simulink model "Hornet_6DOF_FlightSim"  (R2026b)
settings: Solver=VariableStepAuto  StopTime=25.0
values from neighbouring files (symbols this model uses):
  F_g_I = [-weight;0;0]    [Hornet_6DOF_FS_init.m]
  g = 9.81    [Hornet_6DOF_FS_init.m]    (also in hornet_sim_1D_init.m)
  gimbal_max = deg2rad(8)    [Hornet_6DOF_FS_init.m]
  I = [1 0 0 ... (first row only)    [Hornet_6DOF_FS_init.m]
  L_EDF = 1    [Hornet_6DOF_FS_init.m]
  m = 100    [Hornet_6DOF_FS_init.m]    (also in hornet_sim_1D_init.m = 2)
  PID_KD_pitch = 4.0    (= 4)    [Hornet_6DOF_FS_init.m]
  PID_KD_yaw = 4.0    (= 4)    [Hornet_6DOF_FS_init.m]
  PID_KI_pitch = 0.0    (= 0)    [Hornet_6DOF_FS_init.m]
  PID_KI_yaw = 0.0    (= 0)    [Hornet_6DOF_FS_init.m]
  PID_KP_pitch = 4.0    (= 4)    [Hornet_6DOF_FS_init.m]
  PID_KP_yaw = 4.0    (= 4)    [Hornet_6DOF_FS_init.m]
  PIDX_KD_pos = 0.0    (= 0)    [Hornet_6DOF_FS_init.m]
  PIDX_KI_pos = 0.0    (= 0)    [Hornet_6DOF_FS_init.m]
  PIDX_KP_pos = 0.0    (= 0)    [Hornet_6DOF_FS_init.m]
  PIDY_KD_pos = 0.6    [Hornet_6DOF_FS_init.m]
  PIDY_KI_pos = 0.0    (= 0)    [Hornet_6DOF_FS_init.m]
  PIDY_KP_pos = 0.2    [Hornet_6DOF_FS_init.m]
  PIDZ_KD_pos = 0.05    [Hornet_6DOF_FS_init.m]
  PIDZ_KD_vel = 0.0    (= 0)    [Hornet_6DOF_FS_init.m]
  PIDZ_KI_pos = 0.0    (= 0)    [Hornet_6DOF_FS_init.m]
  PIDZ_KI_vel = 0.0    (= 0)    [Hornet_6DOF_FS_init.m]
  PIDZ_KP_pos = 0.4    [Hornet_6DOF_FS_init.m]
  PIDZ_KP_vel = 1.0    (= 1)    [Hornet_6DOF_FS_init.m]
  Position_Target_inertial = [x_targ; y_targ;z_targ]    [Hornet_6DOF_FS_init.m]
  vx0 = 0    [Hornet_6DOF_FS_init.m]    (also in hornet_sim_1D_init.m)
  vy0 = 0    [Hornet_6DOF_FS_init.m]
  vz0 = 0    [Hornet_6DOF_FS_init.m]
  x0 = 0    [Hornet_6DOF_FS_init.m]    (also in hornet_sim_1D_init.m = 1)
  x_hat_body = [1;0;0]    [Hornet_6DOF_FS_init.m]
  y0 = 0    [Hornet_6DOF_FS_init.m]
  z0 = 0    [Hornet_6DOF_FS_init.m]
undefined symbols (not defined in the file or in its folder): DiscIntNeverNeededParam
libraries: slpidlib x5, matrix_library x1, sharedutil x1, aerolibutil x1
settings Model: Creator=11and  LastModifiedBy=jet
settings RTWCC: GenCodeOnly=on
settings SimscapeCC: SimscapeLogType=all  SimscapeNominalValues="[{\"value\":\"1\",\"unit\":\"A\"},{\"value\":\"1\",\"unit\":\"bar\"},{\"value\":\"1\",\"unit\":\"cm^2\"},{\"value\":\"1\",\"unit\":\"cm^3/s\"},{\"value\":\"1\",\"unit\":\"kJ/kg\"},{\"value\":\"1\",\"unit\":\"kW\"},{\"value\":\"1\",\"unit\":\"l\"},{\"value\":\"1\",\"unit\":\"N\"},{\"value\":\"1\",\"unit\":\"N*m\"},{\"value\":\"1\",\"unit\":\"V\"},{\"value\":\"0.001\",\"unit\":\"Wb\"}]"

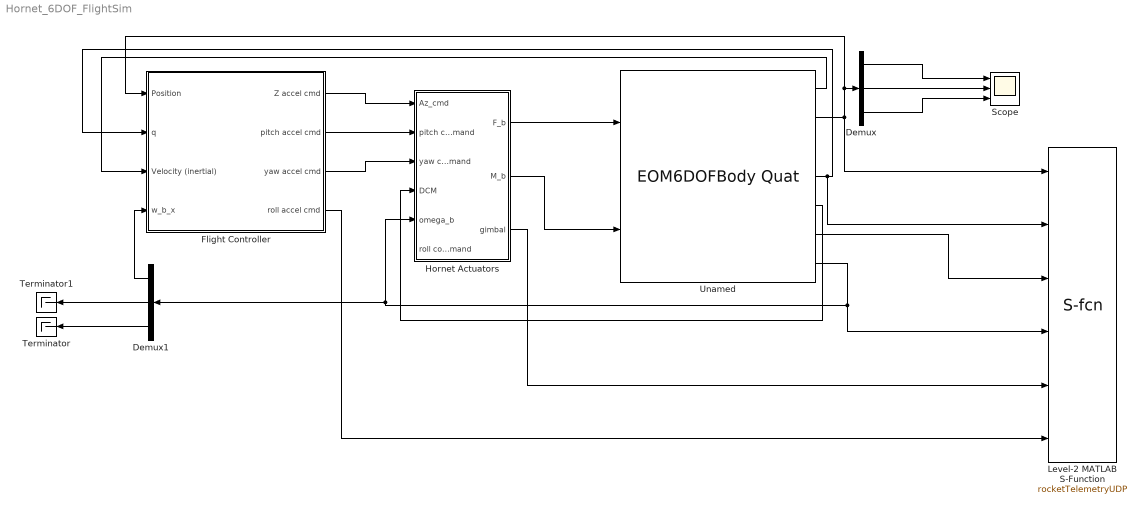
== system Hornet_6DOF_FlightSim ==
  Demux : Demux  Outputs=3
  Demux1 : Demux  Outputs=3
  Flight Controller : Subsystem
  Hornet Actuators : Subsystem
  Level-2 MATLAB S-Function : M-S-Function  FunctionName=rocketTelemetryUDP
      mask Display:
      | port_label('input', 1, 'position_e');
      | port_label('input', 2, 'quaternion_eb');
      | port_label('input', 3, 'velocity_b');
      | port_label('input', 4, 'omega_b');
      | port_label('input', 5, 'gimbal');
      | port_label('input', 6, 'rcs');
  Scope : Scope  NumInputPorts=3
      settings: ActiveDisplayYMinimum=-236.81123475820692  ActiveDisplayYMaximum=587.41234905749616
  Terminator : Terminator
  Terminator1 : Terminator
  Unamed : EOM6DOFBodyQuat  xme_0=[x0 y0 z0]  Vm_0=[vx0 vy0 vz0]  mass_0=m  inertia=I
  wires:
  Unamed/5 -> Hornet Actuators/4(DCM)
  Unamed/2 -> Level-2 MATLAB S-Function/1, Flight Controller/1(Position), Demux/1
  Demux/1 -> Scope/1
  Demux/2 -> Scope/2
  Demux/3 -> Scope/3
  Unamed/4 -> Level-2 MATLAB S-Function/2, Flight Controller/2(q)
  Flight Controller/1(Z accel cmd) -> Hornet Actuators/1(Az_cmd)
  Flight Controller/2(pitch accel cmd) -> Hornet Actuators/2(pitch command)
  Flight Controller/3(yaw accel cmd) -> Hornet Actuators/3(yaw command)
  Hornet Actuators/2(M_b) -> Unamed/2
  Hornet Actuators/1(F_b) -> Unamed/1
  Unamed/7 -> Level-2 MATLAB S-Function/4, Hornet Actuators/5(omega_b), Demux1/1
  Unamed/1 -> Flight Controller/3(Velocity (inertial))
  Demux1/3 -> Terminator/1
  Demux1/2 -> Terminator1/1
  Demux1/1 -> Flight Controller/4(w_b_x)
  Unamed/6 -> Level-2 MATLAB S-Function/3
  Flight Controller/4(roll accel cmd) -> Level-2 MATLAB S-Function/6
  Hornet Actuators/3(gimbal) -> Level-2 MATLAB S-Function/5

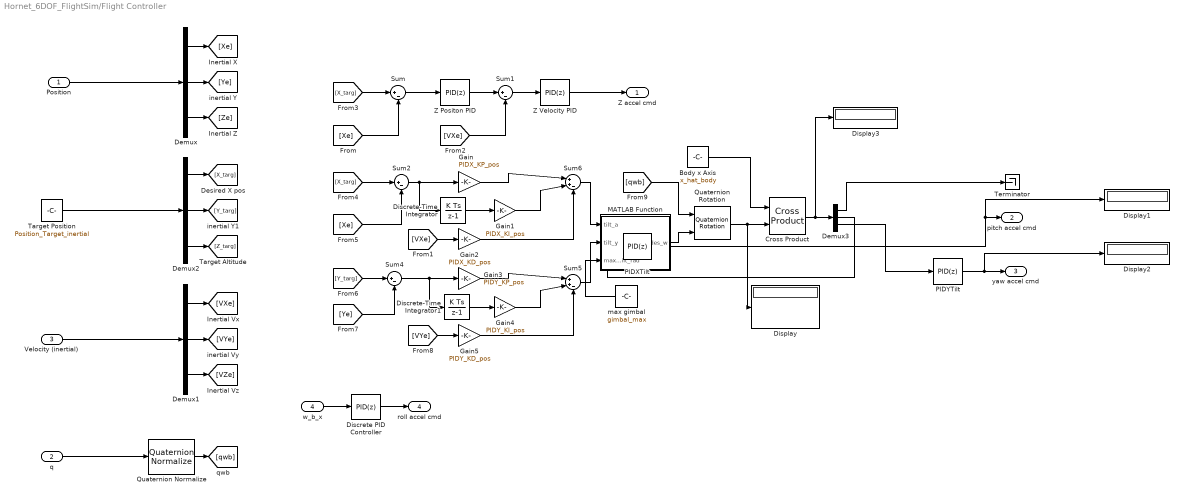
== system Hornet_6DOF_FlightSim/Flight Controller ==
  Position : Inport
  q : Inport  Port=2
  Velocity (inertial) : Inport  Port=3
  w_b_x : Inport  Port=4
  Body x Axis : Constant  Value=x_hat_body
  Cross Product : matrix_library/Cross Product
  Demux{,1..3} (4 alike) : Demux  Outputs=3
  Discrete PID Controller : slpidlib/PID Controller  Controller=PID  Form=Parallel  TimeDomain=Discrete-time  UseExternalTs=off  SampleTime=-1  IntegratorMethod=Forward Euler  FilterMethod=Forward Euler  ControllerParametersSource=internal  P=1  I=1  UseKiTs=off  D=0  UseExternalDerivativeSource=off  N=100  UseFilter=on  TunerSelectOption=Transfer Function Based (PID Tuner App)  InitialConditionSource=internal  InitialConditionForIntegrator=0  InitialConditionForFilter=0  DifferentiatorICPrevScaledInput=0  ExternalReset=none  TrackingMode=off  Kt=1  LimitOutput=off  SatLimitsSource=internal  UpperSaturationLimit=inf  LowerSaturationLimit=-inf  LinearizeAsGain=off  AntiWindupMode=none  Kb=1  LimitIntegrator=off  UpperIntegratorSaturationLimit=inf  LowerIntegratorSaturationLimit=-inf  POutMin=[]  POutMax=[]  IOutMin=[]  IOutMax=[]  DOutMin=[]  DOutMax=[]  NOutMin=[]  NOutMax=[]  SumOutMin=[]  SumOutMax=[]  SaturationOutMin=[]  SaturationOutMax=[]  PParamMin=[]  PParamMax=[]  IParamMin=[]  IParamMax=[]  DParamMin=[]  DParamMax=[]  NParamMin=[]  NParamMax=[]  KbParamMin=[]  KbParamMax=[]  KtParamMin=[]  KtParamMax=[]  KbOutMin=[]  KbOutMax=[]  KtOutMin=[]  KtOutMax=[]  IntegratorOutMin=[]  IntegratorOutMax=[]  FilterOutMin=[]  FilterOutMax=[]  SumI1OutMin=[]  SumI1OutMax=[]  SumI2OutMin=[]  SumI2OutMax=[]  SumI3OutMin=[]  SumI3OutMax=[]  SumI4OutMin=[]  SumI4OutMax=[]  SumDOutMin=[]  SumDOutMax=[]  DifferentiatorOutMin=[]  DifferentiatorOutMax=[]  FilterDiffOutCoefMin=[]  FilterDiffOutCoefMax=[]  ReciprocalOutMin=[]  ReciprocalOutMax=[]  SumDenOutMin=[]  SumDenOutMax=[]  SumNumOutMin=[]  SumNumOutMax=[]  DivideOutMin=[]  DivideOutMax=[]  UdiffTsProdOutMin=[]  UdiffTsProdOutMax=[]  NTsProdOutMin=[]  NTsProdOutMax=[]  UintegralTsProdOutMin=[]  UintegralTsProdOutMax=[]  UngainTsProdOutMin=[]  UngainTsProdOutMax=[]  ClampingZeroOutDataTypeStr=Inherit: Inherit via back propagation  ClampingZeroOutMin=[]  ClampingZeroOutMax=[]  FilterDenConstantOutDataTypeStr=Inherit: Inherit via back propagation  FilterDenConstantOutMin=[]  FilterDenConstantOutMax=[]  PCopyOutDataTypeStr=Inherit: Inherit via back propagation  PCopyOutMin=[]  PCopyOutMax=[]  NCopyOutDataTypeStr=Inherit: Inherit via back propagation  NCopyOutMin=[]  NCopyOutMax=[]  IntegratorContinuousStateAttributes=''  IntegratorStateMustResolveToSignalObject=off  IntegratorRTWStateStorageClass=Auto  FilterContinuousStateAttributes=''  FilterStateMustResolveToSignalObject=off  FilterRTWStateStorageClass=Auto  ParallelPVariant=InternalParameters  IdealPVariant=Disabled  IVariant=InternalParameters  DVariant=InternalParameters  IntegratorVariant=Discrete  SatVariant=Disabled  AWVariant=Passthrough  PCopyVariant=Disabled  TRVariant=Disabled  FdbkBlocksVariant=Forward  IdealPFdbkVariant=Disabled  SatFdbkVariant=Disabled  DerivativeFilterVariant=ForwardEulerFilter  NVariant=InternalParameters  NCopyVariant=Disabled  FilterICVariant=InternalICsFilter  IntegratorICVariant=InternalICs  ExternalResetVariant=Disabled  TRSumVariant=Passthrough  SumFdbkVariant=Disabled  SumVariant=Sum_PID  TsampFilterVariant=InternalTs  TsampNgainVariant=Passthrough  TsampIntegralVariant=Disabled_SignalSpec  ExternalSaturationOutDataTypeStr=Inherit: Same as second input  DerivativeSourceVariant=ErrorSignal  PreIntVariant=InternalPreInt
      settings: LibrarySourceBlock=simulink/Discrete/Discrete PID Controller
  Discrete-Time Integrator : DiscreteIntegrator  SampleTime=-1  ICPrevOutput=DiscIntNeverNeededParam  ICPrevScaledInput=DiscIntNeverNeededParam
  Discrete-Time Integrator1 : DiscreteIntegrator  SampleTime=-1  ICPrevOutput=DiscIntNeverNeededParam  ICPrevScaledInput=DiscIntNeverNeededParam
  Display{,1..3} (4 alike) : Display
  Gain : Gain  Gain=PIDX_KP_pos
  Gain1 : Gain  Gain=PIDX_KI_pos
  Gain2 : Gain  Gain=PIDX_KD_pos
  Gain3 : Gain  Gain=PIDY_KP_pos
  Gain4 : Gain  Gain=PIDY_KI_pos
  Gain5 : Gain  Gain=PIDY_KD_pos
  MATLAB Function : MATLAB Function  TreatAsAtomicUnit=on
  PIDXTilt : slpidlib/PID Controller  Controller=PID  Form=Parallel  TimeDomain=Discrete-time  UseExternalTs=off  SampleTime=-1  IntegratorMethod=Forward Euler  FilterMethod=Forward Euler  ControllerParametersSource=internal  P=PID_KP_pitch  I=PID_KI_pitch  UseKiTs=off  D=PID_KD_pitch  UseExternalDerivativeSource=off  N=100  UseFilter=on  TunerSelectOption=Transfer Function Based (PID Tuner App)  InitialConditionSource=internal  InitialConditionForIntegrator=0  InitialConditionForFilter=0  DifferentiatorICPrevScaledInput=0  ExternalReset=none  TrackingMode=off  Kt=1  LimitOutput=off  SatLimitsSource=internal  UpperSaturationLimit=inf  LowerSaturationLimit=-inf  LinearizeAsGain=off  AntiWindupMode=none  Kb=1  LimitIntegrator=off  UpperIntegratorSaturationLimit=inf  LowerIntegratorSaturationLimit=-inf  POutMin=[]  POutMax=[]  IOutMin=[]  IOutMax=[]  DOutMin=[]  DOutMax=[]  NOutMin=[]  NOutMax=[]  SumOutMin=[]  SumOutMax=[]  SaturationOutMin=[]  SaturationOutMax=[]  PParamMin=[]  PParamMax=[]  IParamMin=[]  IParamMax=[]  DParamMin=[]  DParamMax=[]  NParamMin=[]  NParamMax=[]  KbParamMin=[]  KbParamMax=[]  KtParamMin=[]  KtParamMax=[]  KbOutMin=[]  KbOutMax=[]  KtOutMin=[]  KtOutMax=[]  IntegratorOutMin=[]  IntegratorOutMax=[]  FilterOutMin=[]  FilterOutMax=[]  SumI1OutMin=[]  SumI1OutMax=[]  SumI2OutMin=[]  SumI2OutMax=[]  SumI3OutMin=[]  SumI3OutMax=[]  SumI4OutMin=[]  SumI4OutMax=[]  SumDOutMin=[]  SumDOutMax=[]  DifferentiatorOutMin=[]  DifferentiatorOutMax=[]  FilterDiffOutCoefMin=[]  FilterDiffOutCoefMax=[]  ReciprocalOutMin=[]  ReciprocalOutMax=[]  SumDenOutMin=[]  SumDenOutMax=[]  SumNumOutMin=[]  SumNumOutMax=[]  DivideOutMin=[]  DivideOutMax=[]  UdiffTsProdOutMin=[]  UdiffTsProdOutMax=[]  NTsProdOutMin=[]  NTsProdOutMax=[]  UintegralTsProdOutMin=[]  UintegralTsProdOutMax=[]  UngainTsProdOutMin=[]  UngainTsProdOutMax=[]  ClampingZeroOutDataTypeStr=Inherit: Inherit via back propagation  ClampingZeroOutMin=[]  ClampingZeroOutMax=[]  FilterDenConstantOutDataTypeStr=Inherit: Inherit via back propagation  FilterDenConstantOutMin=[]  FilterDenConstantOutMax=[]  PCopyOutDataTypeStr=Inherit: Inherit via back propagation  PCopyOutMin=[]  PCopyOutMax=[]  NCopyOutDataTypeStr=Inherit: Inherit via back propagation  NCopyOutMin=[]  NCopyOutMax=[]  IntegratorContinuousStateAttributes=''  IntegratorStateMustResolveToSignalObject=off  IntegratorRTWStateStorageClass=Auto  FilterContinuousStateAttributes=''  FilterStateMustResolveToSignalObject=off  FilterRTWStateStorageClass=Auto  ParallelPVariant=InternalParameters  IdealPVariant=Disabled  IVariant=InternalParameters  DVariant=InternalParameters  IntegratorVariant=Discrete  SatVariant=Disabled  AWVariant=Passthrough  PCopyVariant=Disabled  TRVariant=Disabled  FdbkBlocksVariant=Forward  IdealPFdbkVariant=Disabled  SatFdbkVariant=Disabled  DerivativeFilterVariant=ForwardEulerFilter  NVariant=InternalParameters  NCopyVariant=Disabled  FilterICVariant=InternalICsFilter  IntegratorICVariant=InternalICs  ExternalResetVariant=Disabled  TRSumVariant=Passthrough  SumFdbkVariant=Disabled  SumVariant=Sum_PID  TsampFilterVariant=InternalTs  TsampNgainVariant=Passthrough  TsampIntegralVariant=Disabled_SignalSpec  ExternalSaturationOutDataTypeStr=Inherit: Same as second input  DerivativeSourceVariant=ErrorSignal  PreIntVariant=InternalPreInt
      settings: LibrarySourceBlock=simulink/Discrete/Discrete PID Controller
  PIDYTilt : slpidlib/PID Controller  Controller=PID  Form=Parallel  TimeDomain=Discrete-time  UseExternalTs=off  SampleTime=-1  IntegratorMethod=Forward Euler  FilterMethod=Forward Euler  ControllerParametersSource=internal  P=PID_KP_yaw  I=PID_KI_yaw  UseKiTs=off  D=PID_KD_yaw  UseExternalDerivativeSource=off  N=100  UseFilter=on  TunerSelectOption=Transfer Function Based (PID Tuner App)  InitialConditionSource=internal  InitialConditionForIntegrator=0  InitialConditionForFilter=0  DifferentiatorICPrevScaledInput=0  ExternalReset=none  TrackingMode=off  Kt=1  LimitOutput=off  SatLimitsSource=internal  UpperSaturationLimit=inf  LowerSaturationLimit=-inf  LinearizeAsGain=off  AntiWindupMode=none  Kb=1  LimitIntegrator=off  UpperIntegratorSaturationLimit=inf  LowerIntegratorSaturationLimit=-inf  POutMin=[]  POutMax=[]  IOutMin=[]  IOutMax=[]  DOutMin=[]  DOutMax=[]  NOutMin=[]  NOutMax=[]  SumOutMin=[]  SumOutMax=[]  SaturationOutMin=[]  SaturationOutMax=[]  PParamMin=[]  PParamMax=[]  IParamMin=[]  IParamMax=[]  DParamMin=[]  DParamMax=[]  NParamMin=[]  NParamMax=[]  KbParamMin=[]  KbParamMax=[]  KtParamMin=[]  KtParamMax=[]  KbOutMin=[]  KbOutMax=[]  KtOutMin=[]  KtOutMax=[]  IntegratorOutMin=[]  IntegratorOutMax=[]  FilterOutMin=[]  FilterOutMax=[]  SumI1OutMin=[]  SumI1OutMax=[]  SumI2OutMin=[]  SumI2OutMax=[]  SumI3OutMin=[]  SumI3OutMax=[]  SumI4OutMin=[]  SumI4OutMax=[]  SumDOutMin=[]  SumDOutMax=[]  DifferentiatorOutMin=[]  DifferentiatorOutMax=[]  FilterDiffOutCoefMin=[]  FilterDiffOutCoefMax=[]  ReciprocalOutMin=[]  ReciprocalOutMax=[]  SumDenOutMin=[]  SumDenOutMax=[]  SumNumOutMin=[]  SumNumOutMax=[]  DivideOutMin=[]  DivideOutMax=[]  UdiffTsProdOutMin=[]  UdiffTsProdOutMax=[]  NTsProdOutMin=[]  NTsProdOutMax=[]  UintegralTsProdOutMin=[]  UintegralTsProdOutMax=[]  UngainTsProdOutMin=[]  UngainTsProdOutMax=[]  ClampingZeroOutDataTypeStr=Inherit: Inherit via back propagation  ClampingZeroOutMin=[]  ClampingZeroOutMax=[]  FilterDenConstantOutDataTypeStr=Inherit: Inherit via back propagation  FilterDenConstantOutMin=[]  FilterDenConstantOutMax=[]  PCopyOutDataTypeStr=Inherit: Inherit via back propagation  PCopyOutMin=[]  PCopyOutMax=[]  NCopyOutDataTypeStr=Inherit: Inherit via back propagation  NCopyOutMin=[]  NCopyOutMax=[]  IntegratorContinuousStateAttributes=''  IntegratorStateMustResolveToSignalObject=off  IntegratorRTWStateStorageClass=Auto  FilterContinuousStateAttributes=''  FilterStateMustResolveToSignalObject=off  FilterRTWStateStorageClass=Auto  ParallelPVariant=InternalParameters  IdealPVariant=Disabled  IVariant=InternalParameters  DVariant=InternalParameters  IntegratorVariant=Discrete  SatVariant=Disabled  AWVariant=Passthrough  PCopyVariant=Disabled  TRVariant=Disabled  FdbkBlocksVariant=Forward  IdealPFdbkVariant=Disabled  SatFdbkVariant=Disabled  DerivativeFilterVariant=ForwardEulerFilter  NVariant=InternalParameters  NCopyVariant=Disabled  FilterICVariant=InternalICsFilter  IntegratorICVariant=InternalICs  ExternalResetVariant=Disabled  TRSumVariant=Passthrough  SumFdbkVariant=Disabled  SumVariant=Sum_PID  TsampFilterVariant=InternalTs  TsampNgainVariant=Passthrough  TsampIntegralVariant=Disabled_SignalSpec  ExternalSaturationOutDataTypeStr=Inherit: Same as second input  DerivativeSourceVariant=ErrorSignal  PreIntVariant=InternalPreInt
      settings: LibrarySourceBlock=simulink/Discrete/Discrete PID Controller
  Quaternion Normalize : sharedutil/Quaternion Normalize  aMode=aMode
  Quaternion Rotation : aerolibutil/Quaternion Rotation
  Sum{,1..2,4} (4 alike) : Sum  Inputs=|+-
  Sum5 : Sum  Inputs=|++-
  Sum6 : Sum  Inputs=|++-
  Target Position : Constant  Value=Position_Target_inertial
  Terminator : Terminator
  Z Positon PID : slpidlib/PID Controller  Controller=PID  Form=Parallel  TimeDomain=Discrete-time  UseExternalTs=off  SampleTime=-1  IntegratorMethod=Forward Euler  FilterMethod=Forward Euler  ControllerParametersSource=internal  P=PIDZ_KP_pos  I=PIDZ_KI_pos  UseKiTs=off  D=PIDZ_KD_pos  UseExternalDerivativeSource=off  N=100  UseFilter=on  TunerSelectOption=Transfer Function Based (PID Tuner App)  InitialConditionSource=internal  InitialConditionForIntegrator=0  InitialConditionForFilter=0  DifferentiatorICPrevScaledInput=0  ExternalReset=none  TrackingMode=off  Kt=1  LimitOutput=off  SatLimitsSource=internal  UpperSaturationLimit=inf  LowerSaturationLimit=-inf  LinearizeAsGain=off  AntiWindupMode=none  Kb=1  LimitIntegrator=off  UpperIntegratorSaturationLimit=inf  LowerIntegratorSaturationLimit=-inf  POutMin=[]  POutMax=[]  IOutMin=[]  IOutMax=[]  DOutMin=[]  DOutMax=[]  NOutMin=[]  NOutMax=[]  SumOutMin=[]  SumOutMax=[]  SaturationOutMin=[]  SaturationOutMax=[]  PParamMin=[]  PParamMax=[]  IParamMin=[]  IParamMax=[]  DParamMin=[]  DParamMax=[]  NParamMin=[]  NParamMax=[]  KbParamMin=[]  KbParamMax=[]  KtParamMin=[]  KtParamMax=[]  KbOutMin=[]  KbOutMax=[]  KtOutMin=[]  KtOutMax=[]  IntegratorOutMin=[]  IntegratorOutMax=[]  FilterOutMin=[]  FilterOutMax=[]  SumI1OutMin=[]  SumI1OutMax=[]  SumI2OutMin=[]  SumI2OutMax=[]  SumI3OutMin=[]  SumI3OutMax=[]  SumI4OutMin=[]  SumI4OutMax=[]  SumDOutMin=[]  SumDOutMax=[]  DifferentiatorOutMin=[]  DifferentiatorOutMax=[]  FilterDiffOutCoefMin=[]  FilterDiffOutCoefMax=[]  ReciprocalOutMin=[]  ReciprocalOutMax=[]  SumDenOutMin=[]  SumDenOutMax=[]  SumNumOutMin=[]  SumNumOutMax=[]  DivideOutMin=[]  DivideOutMax=[]  UdiffTsProdOutMin=[]  UdiffTsProdOutMax=[]  NTsProdOutMin=[]  NTsProdOutMax=[]  UintegralTsProdOutMin=[]  UintegralTsProdOutMax=[]  UngainTsProdOutMin=[]  UngainTsProdOutMax=[]  ClampingZeroOutDataTypeStr=Inherit: Inherit via back propagation  ClampingZeroOutMin=[]  ClampingZeroOutMax=[]  FilterDenConstantOutDataTypeStr=Inherit: Inherit via back propagation  FilterDenConstantOutMin=[]  FilterDenConstantOutMax=[]  PCopyOutDataTypeStr=Inherit: Inherit via back propagation  PCopyOutMin=[]  PCopyOutMax=[]  NCopyOutDataTypeStr=Inherit: Inherit via back propagation  NCopyOutMin=[]  NCopyOutMax=[]  IntegratorContinuousStateAttributes=''  IntegratorStateMustResolveToSignalObject=off  IntegratorRTWStateStorageClass=Auto  FilterContinuousStateAttributes=''  FilterStateMustResolveToSignalObject=off  FilterRTWStateStorageClass=Auto  ParallelPVariant=InternalParameters  IdealPVariant=Disabled  IVariant=InternalParameters  DVariant=InternalParameters  IntegratorVariant=Discrete  SatVariant=Disabled  AWVariant=Passthrough  PCopyVariant=Disabled  TRVariant=Disabled  FdbkBlocksVariant=Forward  IdealPFdbkVariant=Disabled  SatFdbkVariant=Disabled  DerivativeFilterVariant=ForwardEulerFilter  NVariant=InternalParameters  NCopyVariant=Disabled  FilterICVariant=InternalICsFilter  IntegratorICVariant=InternalICs  ExternalResetVariant=Disabled  TRSumVariant=Passthrough  SumFdbkVariant=Disabled  SumVariant=Sum_PID  TsampFilterVariant=InternalTs  TsampNgainVariant=Passthrough  TsampIntegralVariant=Disabled_SignalSpec  ExternalSaturationOutDataTypeStr=Inherit: Same as second input  DerivativeSourceVariant=ErrorSignal  PreIntVariant=InternalPreInt
      settings: LibrarySourceBlock=simulink/Discrete/Discrete PID Controller
  Z Velocity PID : slpidlib/PID Controller  Controller=PID  Form=Parallel  TimeDomain=Discrete-time  UseExternalTs=off  SampleTime=-1  IntegratorMethod=Forward Euler  FilterMethod=Forward Euler  ControllerParametersSource=internal  P=PIDZ_KP_vel  I=PIDZ_KI_vel  UseKiTs=off  D=PIDZ_KD_vel  UseExternalDerivativeSource=off  N=100  UseFilter=on  TunerSelectOption=Transfer Function Based (PID Tuner App)  InitialConditionSource=internal  InitialConditionForIntegrator=0  InitialConditionForFilter=0  DifferentiatorICPrevScaledInput=0  ExternalReset=none  TrackingMode=off  Kt=1  LimitOutput=off  SatLimitsSource=internal  UpperSaturationLimit=inf  LowerSaturationLimit=-inf  LinearizeAsGain=off  AntiWindupMode=none  Kb=1  LimitIntegrator=off  UpperIntegratorSaturationLimit=inf  LowerIntegratorSaturationLimit=-inf  POutMin=[]  POutMax=[]  IOutMin=[]  IOutMax=[]  DOutMin=[]  DOutMax=[]  NOutMin=[]  NOutMax=[]  SumOutMin=[]  SumOutMax=[]  SaturationOutMin=[]  SaturationOutMax=[]  PParamMin=[]  PParamMax=[]  IParamMin=[]  IParamMax=[]  DParamMin=[]  DParamMax=[]  NParamMin=[]  NParamMax=[]  KbParamMin=[]  KbParamMax=[]  KtParamMin=[]  KtParamMax=[]  KbOutMin=[]  KbOutMax=[]  KtOutMin=[]  KtOutMax=[]  IntegratorOutMin=[]  IntegratorOutMax=[]  FilterOutMin=[]  FilterOutMax=[]  SumI1OutMin=[]  SumI1OutMax=[]  SumI2OutMin=[]  SumI2OutMax=[]  SumI3OutMin=[]  SumI3OutMax=[]  SumI4OutMin=[]  SumI4OutMax=[]  SumDOutMin=[]  SumDOutMax=[]  DifferentiatorOutMin=[]  DifferentiatorOutMax=[]  FilterDiffOutCoefMin=[]  FilterDiffOutCoefMax=[]  ReciprocalOutMin=[]  ReciprocalOutMax=[]  SumDenOutMin=[]  SumDenOutMax=[]  SumNumOutMin=[]  SumNumOutMax=[]  DivideOutMin=[]  DivideOutMax=[]  UdiffTsProdOutMin=[]  UdiffTsProdOutMax=[]  NTsProdOutMin=[]  NTsProdOutMax=[]  UintegralTsProdOutMin=[]  UintegralTsProdOutMax=[]  UngainTsProdOutMin=[]  UngainTsProdOutMax=[]  ClampingZeroOutDataTypeStr=Inherit: Inherit via back propagation  ClampingZeroOutMin=[]  ClampingZeroOutMax=[]  FilterDenConstantOutDataTypeStr=Inherit: Inherit via back propagation  FilterDenConstantOutMin=[]  FilterDenConstantOutMax=[]  PCopyOutDataTypeStr=Inherit: Inherit via back propagation  PCopyOutMin=[]  PCopyOutMax=[]  NCopyOutDataTypeStr=Inherit: Inherit via back propagation  NCopyOutMin=[]  NCopyOutMax=[]  IntegratorContinuousStateAttributes=''  IntegratorStateMustResolveToSignalObject=off  IntegratorRTWStateStorageClass=Auto  FilterContinuousStateAttributes=''  FilterStateMustResolveToSignalObject=off  FilterRTWStateStorageClass=Auto  ParallelPVariant=InternalParameters  IdealPVariant=Disabled  IVariant=InternalParameters  DVariant=InternalParameters  IntegratorVariant=Discrete  SatVariant=Disabled  AWVariant=Passthrough  PCopyVariant=Disabled  TRVariant=Disabled  FdbkBlocksVariant=Forward  IdealPFdbkVariant=Disabled  SatFdbkVariant=Disabled  DerivativeFilterVariant=ForwardEulerFilter  NVariant=InternalParameters  NCopyVariant=Disabled  FilterICVariant=InternalICsFilter  IntegratorICVariant=InternalICs  ExternalResetVariant=Disabled  TRSumVariant=Passthrough  SumFdbkVariant=Disabled  SumVariant=Sum_PID  TsampFilterVariant=InternalTs  TsampNgainVariant=Passthrough  TsampIntegralVariant=Disabled_SignalSpec  ExternalSaturationOutDataTypeStr=Inherit: Same as second input  DerivativeSourceVariant=ErrorSignal  PreIntVariant=InternalPreInt
      settings: LibrarySourceBlock=simulink/Discrete/Discrete PID Controller
  max gimbal : Constant  Value=gimbal_max
  Z accel cmd : Outport
  pitch accel cmd : Outport  Port=2
  yaw accel cmd : Outport  Port=3
  roll accel cmd : Outport  Port=4
  wires:
  [X_targ] -> Sum/1
  Sum/1 -> Z Positon PID/1
  Z Velocity PID/1 -> Z accel cmd/1
  Position/1 -> Demux/1
  Demux/1 -> [Xe]
  [Xe] -> Sum/2
  Z Positon PID/1 -> Sum1/1
  Demux1/1 -> [VXe]
  Demux1/2 -> [VYe]
  Demux1/3 -> [VZe]
  [VXe] -> Sum1/2
  Sum1/1 -> Z Velocity PID/1
  Demux2/1 -> [X_targ]
  Demux2/2 -> [Y_targ]
  Demux2/3 -> [Z_targ]
  Sum2/1 -> Discrete-Time Integrator/1, Gain/1
  [X_targ] -> Sum2/1
  [Xe] -> Sum2/2
  [Y_targ] -> Sum4/1
  [Ye] -> Sum4/2
  [VXe] -> Gain2/1
  Gain/1 -> Sum6/1
  Gain2/1 -> Sum6/3
  PIDXTilt/1 -> Display1/1, pitch accel cmd/1
  PIDYTilt/1 -> Display2/1, yaw accel cmd/1
  Gain5/1 -> Sum5/3
  [VYe] -> Gain5/1
  Sum4/1 -> Discrete-Time Integrator1/1, Gain3/1
  Gain3/1 -> Sum5/1
  Sum6/1 -> MATLAB Function/1(tilt_a)
  Sum5/1 -> MATLAB Function/2(tilt_y)
  MATLAB Function/1(z_des_w) -> Quaternion Rotation/2
  Quaternion Rotation/1 -> Display/1, Cross Product/2
  Body x Axis/1 -> Cross Product/1
  Cross Product/1 -> Display3/1, Demux3/1
  [qwb] -> Quaternion Rotation/1
  Demux3/2 -> PIDXTilt/1
  Demux3/1 -> Terminator/1
  Demux3/3 -> PIDYTilt/1
  Demux/2 -> [Ye]
  Demux/3 -> [Ze]
  Target Position/1 -> Demux2/1
  Quaternion Normalize/1 -> [qwb]
  max gimbal/1 -> MATLAB Function/3(max_tilt_rad)
  Discrete-Time Integrator1/1 -> Gain4/1
  Gain4/1 -> Sum5/2
  Discrete-Time Integrator/1 -> Gain1/1
  Gain1/1 -> Sum6/2
  Velocity (inertial)/1 -> Demux1/1
  w_b_x/1 -> Discrete PID Controller/1
  Discrete PID Controller/1 -> roll accel cmd/1
  q/1 -> Quaternion Normalize/1

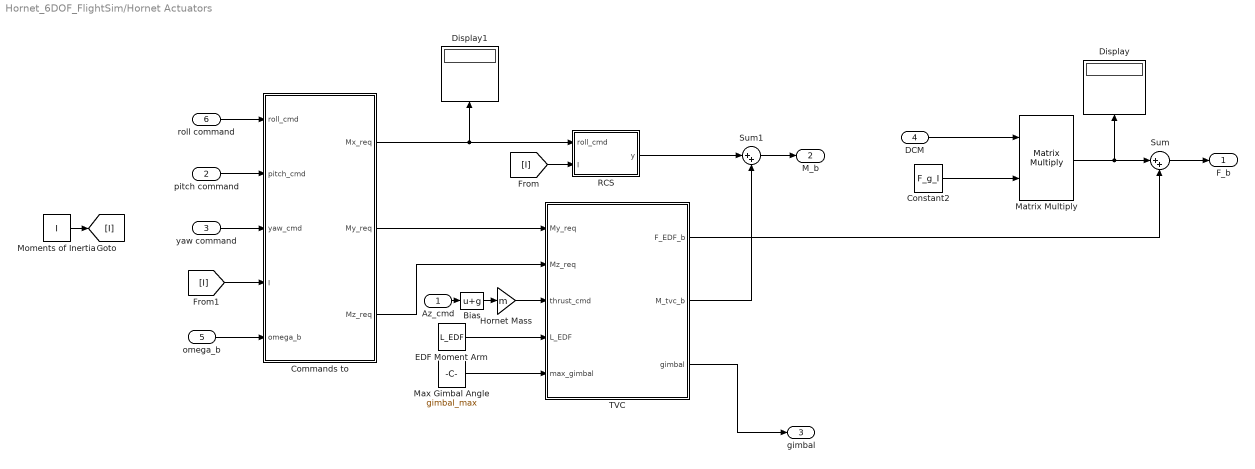
== system Hornet_6DOF_FlightSim/Hornet Actuators ==
  Az_cmd : Inport
  pitch command : Inport  Port=2
  yaw command : Inport  Port=3
  DCM : Inport  Port=4
  omega_b : Inport  Port=5
  roll command : Inport  Port=6
  Bias : Bias  Bias=g  SaturateOnIntegerOverflow=off
  "Commands to " : MATLAB Function  TreatAsAtomicUnit=on
  Constant2 : Constant  Value=F_g_I
  Display : Display
  Display1 : Display
  EDF Moment Arm : Constant  Value=L_EDF
  Hornet Mass : Gain  Gain=m
  Matrix Multiply : Product  Multiplication=Matrix(*)
  Max Gimbal Angle : Constant  Value=gimbal_max
  Moments of Inertia : Constant  Value=I
  RCS : MATLAB Function  TreatAsAtomicUnit=on
  Sum : Sum  Inputs=|++
  Sum1 : Sum  Inputs=|++
  TVC : MATLAB Function  TreatAsAtomicUnit=on
  F_b : Outport
  M_b : Outport  Port=2
  gimbal : Outport  Port=3
  wires:
  Hornet Mass/1 -> TVC/3(thrust_cmd)
  EDF Moment Arm/1 -> TVC/4(L_EDF)
  Constant2/1 -> Matrix Multiply/2
  Matrix Multiply/1 -> Display/1, Sum/1
  Sum/1 -> F_b/1
  "Commands to "/2(My_req) -> TVC/1(My_req)
  yaw command/1 -> "Commands to "/3(yaw_cmd)
  pitch command/1 -> "Commands to "/2(pitch_cmd)
  omega_b/1 -> "Commands to "/5(omega_b)
  "Commands to "/1(Mx_req) -> RCS/1(roll_cmd), Display1/1
  Max Gimbal Angle/1 -> TVC/5(max_gimbal)
  TVC/2(M_tvc_b) -> Sum1/2
  roll command/1 -> "Commands to "/1(roll_cmd)
  "Commands to "/3(Mz_req) -> TVC/2(Mz_req)
  Sum1/1 -> M_b/1
  RCS/1(y) -> Sum1/1
  TVC/1(F_EDF_b) -> Sum/2
  Moments of Inertia/1 -> [I]
  [I] -> RCS/2(I)
  [I] -> "Commands to "/4(I)
  TVC/3(gimbal) -> gimbal/1
  DCM/1 -> Matrix Multiply/1
  Az_cmd/1 -> Bias/1
  Bias/1 -> Hornet Mass/1

== matlab function Hornet_6DOF_FlightSim/Hornet Actuators/TVC ==
  data: My_req input; F_EDF_b output; Mz_req input; thrust_cmd input; L_EDF input; M_tvc_b output; max_gimbal input; gimbal output
function [F_EDF_b, M_tvc_b, gimbal] = fcn(My_req, Mz_req, thrust_cmd, L_EDF, max_gimbal)
L = L_EDF;
%% Eventually, we can add transient properties, that's why these are labeled as required/desired torques

%dy_cmd = My_req / (thrust_cmd * L); % y-rotation gimbal angle from small angle approx
%dz_cmd = Mz_req / (thrust_cmd * L); % z-rotation gimbal angle from small angle approx
dy_cmd = -My_req / (thrust_cmd * L); % JACK: Sign flip
dz_cmd = -Mz_req / (thrust_cmd * L);

dy_cmd = max(min(dy_cmd, max_gimbal), -max_gimbal); % limiting gimbal angles
dz_cmd = max(min(dz_cmd, max_gimbal), -max_gimbal);

u = [cos(dz_cmd)*cos(dy_cmd); sin(dz_cmd)*cos(dy_cmd); -sin(dy_cmd)];
F_EDF_b = thrust_cmd * u;
M_tvc_b = cross([-L;0;0], F_EDF_b); % JACK: F_b -> F_EDF_b

%% The code above is temporary so that I can figure out some bugs
gimbal = [dy_cmd; dz_cmd]; % JACK: added for the viewer

== matlab function Hornet_6DOF_FlightSim/Hornet Actuators/RCS ==
  data: roll_cmd input; y output; I input
% function y = fcn(roll_cmd, I)
% Ixx = I(1,1);
% 
% Mx = 
% y = u;

function y = fcn(roll_cmd, I)
y = zeros(3,1); % JACK: replaced to placeholder so it runs minimally.

== matlab function Hornet_6DOF_FlightSim/Flight Controller/MATLAB Function ==
  data: tilt_a input; z_des_w output; tilt_y input; max_tilt_rad input
function z_des_w = fcn(tilt_a, tilt_y, max_tilt_rad)

%world_tilt_x = clip(world_tilt_x, -max_tilt_rad, max_tilt_rad);
%world_tilt_y = clip(world_tilt_y, -max_tilt_rad, max_tilt_rad);

%z = [tan(world_tilt_x); tan(world_tilt_y); 1];
%z_des_w = z / norm(z);
tilt_a = clip(tilt_a, -max_tilt_rad, max_tilt_rad);
tilt_y = clip(tilt_y, -max_tilt_rad, max_tilt_rad);
z = [1; tan(tilt_y); tan(tilt_a)];
z_des_w = z / norm(z);

end

== matlab function Hornet_6DOF_FlightSim/Hornet Actuators/Commands to  ==
  data: roll_cmd input; pitch_cmd input; Mx_req output; yaw_cmd input; My_req output; I input; omega_b input; Mz_req output
function [Mx_req, My_req, Mz_req]= fcn(roll_cmd, pitch_cmd, yaw_cmd, I, omega_b)
    
    alpha_cmd = [roll_cmd; pitch_cmd; yaw_cmd];
    
    M_b_req = I*alpha_cmd + cross(omega_b, I*omega_b);
    
    Mx_req = M_b_req(1);   
    My_req = M_b_req(2);
    Mz_req = M_b_req(3);
